simulink model "MPCSmallSize"  (R2017a)
settings: Solver=VariableStepAuto  StartTime=0.0  StopTime=10.0  RelTol=1e-3
libraries: dspinverses x1
settings Model: Creator=Pichau  LastModifiedBy=Pichau

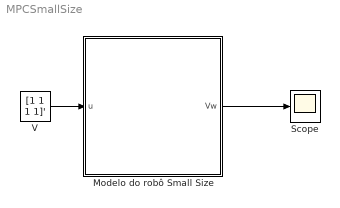
== system MPCSmallSize ==
  Modelo do robô Small Size : Subsystem  mask{R=1, massa=1, raio=1, compr=1, yCM=0, xCM=0, ICM=1, N=1, eta=1, Jm=1, Jw=1, k=1, Bm=1, Bw=1}
      mask prompts: R "Resistência do motor"; massa "Massa do robô"; raio "Raio da roda"; compr "Distância da roda ao CM"; yCM "Y do CM"; xCM "X do CM"; ICM "Momento de inércia em relação ao CM"; N "Redução N"; eta "Eficiência do sistema de redução"; Jm "Inercia do motor Jm"; Jw "Inercia da roda Jw"; k "Constante de torque do motor K"; Bm "Coeficiente de atrito viscoso do motor Bm"; Bw "Coeficiente de atrito viscoso da roda Bw"
      mask Display: image('Glados.png');
  Scope : Scope
  V : Constant  Value=[1 1 1 1]'
  wires:
  V/1 -> Modelo do robô Small Size/1(u)
  Modelo do robô Small Size/1(Vw) -> Scope/1

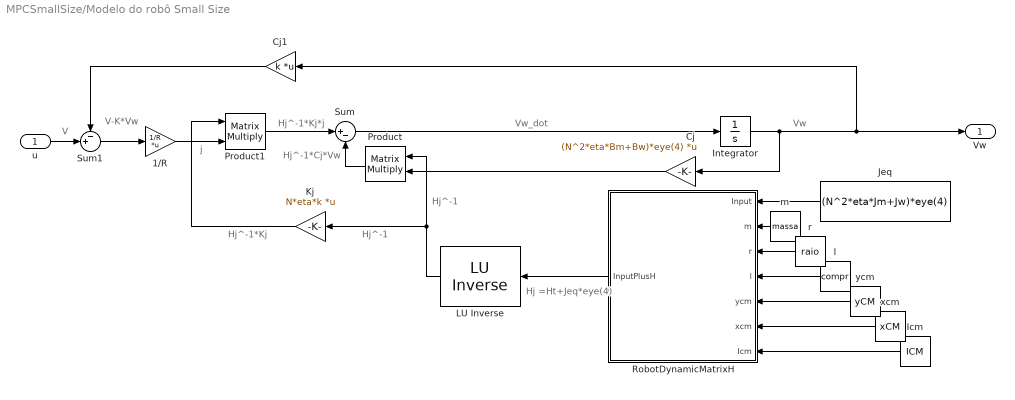
== system MPCSmallSize/Modelo do robô Small Size ==
  note: V-K*Vw
  note: V
  note: Hj^-1*Kj*j
  note: Hj^-1*Cj*Vw
  note: j
  note: Hj =Ht+Jeq*eye(4)
  note: Vw_dot
  note: Vw
  note: Hj^-1
  note: Hj^-1*Kj
  note: Hj^-1
  u : Inport
  " LU Inverse" : dspinverses/ LU Inverse
      settings: SourceProductName=DSP System Toolbox
  1/R : Gain  Gain=1/R  Multiplication=Matrix(K*u)
  Cj : Gain  Gain=(N^2*eta*Bm+Bw)*eye(4)  Multiplication=Matrix(K*u)
  Cj1 : Gain  Gain=k  Multiplication=Matrix(K*u)
  Icm : Constant  Value=ICM
  Integrator : Integrator
  Jeq : Constant  Value=(N^2*eta*Jm+Jw)*eye(4)
  Kj : Gain  Gain=N*eta*k  Multiplication=Matrix(K*u)
  Product : Product  Multiplication=Matrix(*)
  Product1 : Product  Multiplication=Matrix(*)
  RobotDynamicMatrixH : MATLAB Function  TreatAsAtomicUnit=on
  Sum : Sum  Inputs=|+-
  Sum1 : Sum  Inputs=-+|
  l : Constant  Value=compr
  "m " : Constant  Value=massa
  r : Constant  Value=raio
  xcm : Constant  Value=xCM
  ycm : Constant  Value=yCM
  Vw : Outport
  wires:
  ycm/1 -> RobotDynamicMatrixH/5(ycm)
  r/1 -> RobotDynamicMatrixH/3(r)
  xcm/1 -> RobotDynamicMatrixH/6(xcm)
  Sum/1 -> Integrator/1
  l/1 -> RobotDynamicMatrixH/4(l)
  Jeq/1 -> RobotDynamicMatrixH/1(Input)
  Icm/1 -> RobotDynamicMatrixH/7(Icm)
  "m "/1 -> RobotDynamicMatrixH/2(m)
  RobotDynamicMatrixH/1(InputPlusH) -> " LU Inverse"/1
  Product/1 -> Sum/2
  " LU Inverse"/1 -> Kj/1, Product/1
  Integrator/1 -> Cj1/1, Vw/1, Cj/1
  Cj/1 -> Product/2
  Kj/1 -> Product1/1
  Product1/1 -> Sum/1
  Cj1/1 -> Sum1/1
  u/1 -> Sum1/2
  Sum1/1 -> 1/R/1
  1/R/1 -> Product1/2

== matlab function MPCSmallSize/Modelo do robô Small Size/RobotDynamicMatrixH ==
  data: Input input; InputPlusH output; m input; r input; l input; ycm input; xcm input; Icm input
function InputPlusH = RobotDynamicMatrixH(Input,m,r,l,ycm,xcm,Icm)
%#codegen

%    This function was generated by the Symbolic Math Toolbox version 7.2.
%    07-May-2019 23:41:05

t2 = sqrt(2.0);
t3 = 1.0./l.^2;
t4 = r.^2;
t5 = xcm.^2;
t6 = m.*t5;
t7 = ycm.^2;
t8 = m.*t7;
t9 = l.*m.*t2.*ycm.*2.0;
t10 = l.^2;
t11 = m.*t10.*4.0;
t12 = l.*m.*t2.*xcm.*2.0;
t13 = Icm+t6+t8+t9;
t14 = t3.*t4.*t13.*(1.0./1.6e1);
t15 = Icm+t6+t8-t11;
t16 = t3.*t4.*t15.*(1.0./1.6e1);
t17 = Icm+t6+t8-t12;
t18 = t3.*t4.*t17.*(1.0./1.6e1);
t19 = Icm+t6+t8+t12;
t20 = t3.*t4.*t19.*(1.0./1.6e1);
t21 = Icm+t6+t8-t9;
t22 = t3.*t4.*t21.*(1.0./1.6e1);
InputPlusH = reshape([t3.*t4.*(Icm+t6+t8+t9+t11+t12).*(1.0./1.6e1),t14,t16,t20,t14,t3.*t4.*(Icm+t6+t8+t9+t11-t12).*(1.0./1.6e1),t18,t16,t16,t18,t3.*t4.*(Icm+t6+t8-t9+t11-t12).*(1.0./1.6e1),t22,t20,t16,t22,t3.*t4.*(Icm+t6+t8-t9+t11+t12).*(1.0./1.6e1)],[4,4]);
InputPlusH = (InputPlusH + Input);
